simulink subsystem "Kalman_Filter"  (R2019b)
settings: Solver=VariableStepAuto  StartTime=0.0  StopTime=10.0  RelTol=1e-3
undefined symbols (not defined in the file): PF_delay
settings Model: Creator=toons  LastModifiedBy=toons

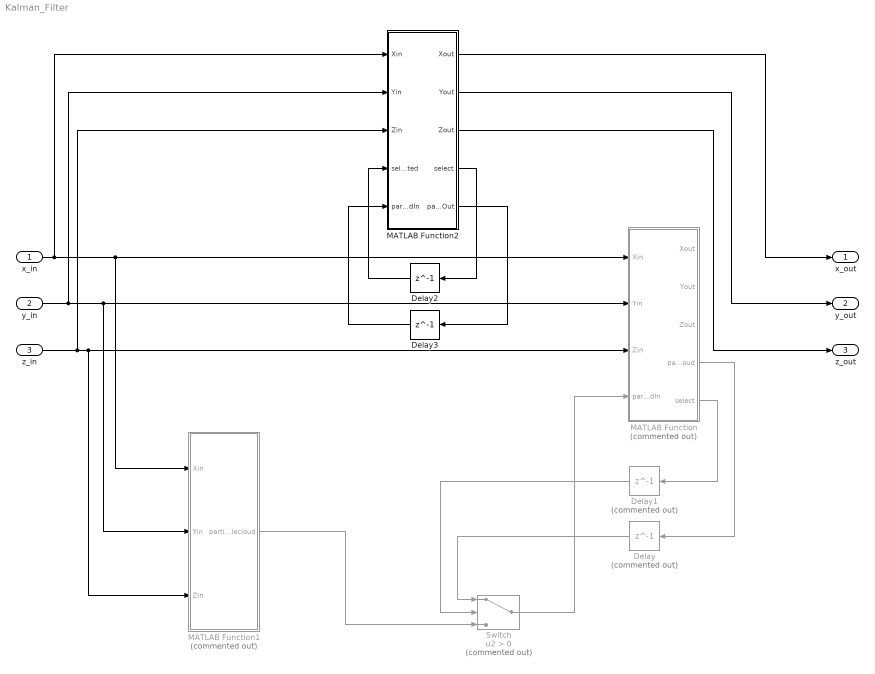
== system Kalman_Filter ==
  x_in : Inport
  y_in : Inport  Port=2
  z_in : Inport  Port=3
  Delay : Delay  Commented=on  DelayLength=1  InitialCondition=0
  Delay1 : Delay  Commented=on  DelayLength=1  InitialCondition=0
  Delay2 : Delay  DelayLength=1  InitialCondition=0  SampleTime=PF_delay
  Delay3 : Delay  DelayLength=1  InitialCondition=0  SampleTime=PF_delay
  MATLAB Function : MATLAB Function  Commented=on  TreatAsAtomicUnit=on
  MATLAB Function1 : MATLAB Function  Commented=on  TreatAsAtomicUnit=on
  MATLAB Function2 : MATLAB Function  TreatAsAtomicUnit=on
  Switch : Switch  Commented=on  Criteria=u2 > Threshold
  x_out : Outport
  y_out : Outport  Port=2
  z_out : Outport  Port=3
  wires:
  y_in/1 -> MATLAB Function1/2(Yin), MATLAB Function/2(Yin), MATLAB Function2/2(Yin)
  x_in/1 -> MATLAB Function1/1(Xin), MATLAB Function/1(Xin), MATLAB Function2/1(Xin)
  z_in/1 -> MATLAB Function1/3(Zin), MATLAB Function/3(Zin), MATLAB Function2/3(Zin)
  MATLAB Function1/1(particlecloud) -> Switch/3
  Switch/1 -> MATLAB Function/4(particlecloudIn)
  MATLAB Function/5(select) -> Delay1/1
  MATLAB Function/4(particlecloud) -> Delay/1
  Delay/1 -> Switch/1
  Delay1/1 -> Switch/2
  MATLAB Function2/1(Xout) -> x_out/1
  MATLAB Function2/2(Yout) -> y_out/1
  MATLAB Function2/3(Zout) -> z_out/1
  MATLAB Function2/4(select) -> Delay2/1
  Delay2/1 -> MATLAB Function2/4(selected)
  MATLAB Function2/5(particlecloudOut) -> Delay3/1
  Delay3/1 -> MATLAB Function2/5(particlecloudIn)

== matlab function Kalman_Filter/MATLAB Function ==
  data: Xin input; Xout output; Yin input; Zin input; Yout output; Zout output; particlecloudIn input; particlecloud output; select output
function [Xout,Yout,Zout, particlecloud, select]= fcn(Xin,Yin,Zin,particlecloudIn)

locationMusquito = [Xin,Yin,Zin];
numberParticles = 500;

xm = locationMusquito(1);
ym = locationMusquito(2);
zm = locationMusquito(3);

measuredPos = locationMusquito;


changeVariationLoc = 0.01;
changeVariationSpeed = 0.01;
changeVariationAngle = 0.4;
changeVariationAcceleration = 0.01;
changeVariationSpeedAngle = 0.1;

particlecloud = particlecloudIn;


    %updateLocation;
    
  particlecloud(:,1) = particlecloud(:,1) + particlecloud(:,4) .* cos(particlecloud(:,5));
  particlecloud(:,2) = particlecloud(:,2) + particlecloud(:,4) .* sin(particlecloud(:,5));
  particlecloud(:,3) = particlecloud(:,3) + particlecloud(:,4) .* sin(particlecloud(:,6));
  particlecloud(:,4) = particlecloud(:,4) + particlecloud(:,7);
  particlecloud(:,5) = particlecloud(:,5) + particlecloud(:,8);
  particlecloud(:,6) = particlecloud(:,6) + particlecloud(:,9);
  particlecloud(:,7) = particlecloud(:,7);
  particlecloud(:,8) = particlecloud(:,8);
  particlecloud(:,9) = particlecloud(:,9);
  
  %L2 difference
  weight = sqrt(measuredPos(1) - particlecloud(:,1)).^2 + (measuredPos(2) - particlecloud(:,2) + (measuredPos(1) - particlecloud(:,1)).^2);
  weight = 1./weight;
  weight = weight ./ sum(weight);
  
  particlecloud(:,24) = particlecloud(:,23);
  particlecloud(:,23) = particlecloud(:,22);
  particlecloud(:,22) = particlecloud(:,21);
  particlecloud(:,21) = particlecloud(:,20);
  particlecloud(:,20) = particlecloud(:,19);
  particlecloud(:,19) = particlecloud(:,18);
  particlecloud(:,18) = particlecloud(:,17);
  particlecloud(:,17) = particlecloud(:,16);
  particlecloud(:,16) = particlecloud(:,15);
  particlecloud(:,15) = particlecloud(:,14);
  particlecloud(:,14) = particlecloud(:,13);
  particlecloud(:,13) = particlecloud(:,12);
  particlecloud(:,12) = particlecloud(:,11);
  particlecloud(:,11) = weight;
  particlecloud(:,10) = (3*particlecloud(:,11)+particlecloud(:,12)+particlecloud(:,13)+particlecloud(:,14)+particlecloud(:,15)+particlecloud(:,16)+particlecloud(:,17)+particlecloud(:,18)+particlecloud(:,19)+particlecloud(:,20)+particlecloud(:,21)+particlecloud(:,22)+particlecloud(:,23)+particlecloud(:,24))./18;
  particlecloud(:,10) = particlecloud(:,10) ./ sum(particlecloud(:,10));
  
  [valueMax indexMax]=max(particlecloud(:,7));
  bestPos = [particlecloud(indexMax,1),particlecloud(indexMax,2), particlecloud(indexMax,3)];
  
  selecting = particlecloud;
  selecting(:,7) = (40*particlecloud(:,8)+particlecloud(:,9)+particlecloud(:,10)+particlecloud(:,11)+particlecloud(:,12)+particlecloud(:,13)+particlecloud(:,14)+particlecloud(:,15)+particlecloud(:,16)+particlecloud(:,17)+particlecloud(:,18)+particlecloud(:,19)+particlecloud(:,20))./14;
  selecting(:,7) = selecting(:,7) ./ sum(selecting(:,7));
  [~,idx] = sort(selecting(:,7)); % sort just the first column
  selecting = selecting(idx,:);   % sort the whole matrix using the sort indices

  for i=1:(numberParticles*0.1)
    particlecloud(i+numberParticles*0.9,:) = selecting(numberParticles-i,:);
  end
  weight = cumsum(weight);
  for i=1:(numberParticles*0.9)
    selecting(i,1) = find(weight >= rand(1),1);
  end
  for i=1:(numberParticles*0.9)
    particlecloud(i,:) = particlecloud(selecting(i,1),:);
        particlecloud(i,1) = particlecloud(i,1) + (rand()*changeVariationLoc - (changeVariationLoc/2));
        particlecloud(i,2) = particlecloud(i,2) + (rand()*changeVariationLoc - (changeVariationLoc/2));
        particlecloud(i,3) = particlecloud(i,3) + (rand()*changeVariationLoc - (changeVariationLoc/2));
        particlecloud(i,4) = particlecloud(i,4) * (rand()*changeVariationSpeed - (changeVariationSpeed/2));
        particlecloud(i,5) = particlecloud(i,5) + (rand()*changeVariationAngle - (changeVariationAngle));
        particlecloud(i,6) = particlecloud(i,6) + (rand()*changeVariationAngle - (changeVariationAngle/2));
        particlecloud(i,7) = particlecloud(i,7) * (rand()*changeVariationAcceleration - (changeVariationAcceleration/2));
        particlecloud(i,8) = particlecloud(i,8) * (rand()*changeVariationSpeedAngle - (changeVariationSpeedAngle/2));
        particlecloud(i,9) = particlecloud(i,9) * (rand()*changeVariationSpeedAngle - (changeVariationSpeedAngle/2));
  end

  select = 1;
Xout = bestPos(1);
Yout = bestPos(2);
Zout = bestPos(3);

== matlab function Kalman_Filter/MATLAB Function1 ==
  data: Xin input; Yin input; Zin input; particlecloud output
function particlecloud = fcn(Xin,Yin,Zin)

locationMusquito = [Xin,Yin,Zin];
numberParticles = 500;

xm = locationMusquito(1);
ym = locationMusquito(2);
zm = locationMusquito(3);

bestPos = locationMusquito;

initialVariationLoc = 0.01;
initialVariationSpeed = 0.01;
initialVariationAngle = 1;
initialVariationAcceleration = 0.01;
initialVariationSpeedAngle = 0.1;

particlecloud = rand(numberParticles,24);

%initial variantion but with avarage zero and then + initial value making
%the initial value the average
particlecloud(:,1) = particlecloud(:,1) * initialVariationLoc - (initialVariationLoc/2) + xm;
particlecloud(:,2) = particlecloud(:,2) * initialVariationLoc - (initialVariationLoc/2) + ym;
particlecloud(:,3) = particlecloud(:,3) * initialVariationLoc - (initialVariationLoc/2) + zm;
% initial variation of speed with zero as the average
particlecloud(:,4) = particlecloud(:,4) * initialVariationSpeed - (initialVariationSpeed/2);
% initial variation of the angle with zero as average
particlecloud(:,5) = particlecloud(:,5) * initialVariationAngle - (initialVariationAngle/2);
particlecloud(:,6) = particlecloud(:,6) * initialVariationAngle - (initialVariationAngle/2);
% initial variation of acceleration with zero as the average
particlecloud(:,7) = particlecloud(:,7) * initialVariationAcceleration - (initialVariationAcceleration/2);
% initial variation of the speed of the angle with zero as average
particlecloud(:,8) = particlecloud(:,8) * initialVariationSpeedAngle - (initialVariationSpeedAngle/2);
particlecloud(:,9) = particlecloud(:,9) * initialVariationSpeedAngle - (initialVariationSpeedAngle/2);
particlecloud(:,10) = 0; % weight
particlecloud(:,11) = 0; % previous weight
particlecloud(:,12) = 0; % the one before and so on
particlecloud(:,13) = 0;
particlecloud(:,14) = 0;
particlecloud(:,15) = 0;
particlecloud(:,16) = 0;
particlecloud(:,17) = 0;
particlecloud(:,18) = 0;
particlecloud(:,19) = 0;
particlecloud(:,20) = 0;
particlecloud(:,21) = 0;
particlecloud(:,22) = 0;
particlecloud(:,23) = 0;
particlecloud(:,24) = 0;

particlecloud = particlecloud;
Xout = bestPos(1);
Yout = bestPos(2);
Zout = bestPos(3);

== matlab function Kalman_Filter/MATLAB Function2 ==
  data: Xin input; Yin input; Zin input; Xout output; selected input; Yout output; Zout output; select output; particlecloudIn input; particlecloudOut output size=[500,24]
function [Xout, Yout, Zout, select, particlecloudOut]= fcn(Xin,Yin,Zin, selected, particlecloudIn)



locationMusquito = [Xin,Yin,Zin];
numberParticles = 500;

particlecloud = rand(numberParticles,24);

particlecloud = particlecloudIn;

xm = locationMusquito(1);
ym = locationMusquito(2);
zm = locationMusquito(3);

bestPos = locationMusquito;

if(selected == 0)

initialVariationLoc = 0.01;
initialVariationSpeed = 0.01;
initialVariationAngle = 1;
initialVariationAcceleration = 0.01;
initialVariationSpeedAngle = 0.1;

particlecloud = rand(numberParticles,24);

%initial variantion but with avarage zero and then + initial value making
%the initial value the average
particlecloud(:,1) = particlecloud(:,1) * initialVariationLoc - (initialVariationLoc/2) + xm;
particlecloud(:,2) = particlecloud(:,2) * initialVariationLoc - (initialVariationLoc/2) + ym;
particlecloud(:,3) = particlecloud(:,3) * initialVariationLoc - (initialVariationLoc/2) + zm;
% initial variation of speed with zero as the average
particlecloud(:,4) = particlecloud(:,4) * initialVariationSpeed - (initialVariationSpeed/2);
% initial variation of the angle with zero as average
particlecloud(:,5) = particlecloud(:,5) * initialVariationAngle - (initialVariationAngle/2);
particlecloud(:,6) = particlecloud(:,6) * initialVariationAngle - (initialVariationAngle/2);
% initial variation of acceleration with zero as the average
particlecloud(:,7) = particlecloud(:,7) * initialVariationAcceleration - (initialVariationAcceleration/2);
% initial variation of the speed of the angle with zero as average
particlecloud(:,8) = particlecloud(:,8) * initialVariationSpeedAngle - (initialVariationSpeedAngle/2);
particlecloud(:,9) = particlecloud(:,9) * initialVariationSpeedAngle - (initialVariationSpeedAngle/2);
particlecloud(:,10) = 0; % weight
particlecloud(:,11) = 0; % previous weight
particlecloud(:,12) = 0; % the one before and so on
particlecloud(:,13) = 0;
particlecloud(:,14) = 0;
particlecloud(:,15) = 0;
particlecloud(:,16) = 0;
particlecloud(:,17) = 0;
particlecloud(:,18) = 0;
particlecloud(:,19) = 0;
particlecloud(:,20) = 0;
particlecloud(:,21) = 0;
particlecloud(:,22) = 0;
particlecloud(:,23) = 0;
particlecloud(:,24) = 0;

particlecloud = particlecloud;


end



measuredPos = locationMusquito;


changeVariationLoc = 0.01;
changeVariationSpeed = 0.01;
changeVariationAngle = 0.4;
changeVariationAcceleration = 0.01;
changeVariationSpeedAngle = 0.1;



    %updateLocation;
    
  particlecloud(:,1) = particlecloud(:,1) + particlecloud(:,4) .* cos(particlecloud(:,5));
  particlecloud(:,2) = particlecloud(:,2) + particlecloud(:,4) .* sin(particlecloud(:,5));
  particlecloud(:,3) = particlecloud(:,3) + particlecloud(:,4) .* sin(particlecloud(:,6));
  particlecloud(:,4) = particlecloud(:,4) + particlecloud(:,7);
  particlecloud(:,5) = particlecloud(:,5) + particlecloud(:,8);
  particlecloud(:,6) = particlecloud(:,6) + particlecloud(:,9);
  particlecloud(:,7) = particlecloud(:,7);
  particlecloud(:,8) = particlecloud(:,8);
  particlecloud(:,9) = particlecloud(:,9);
  
  %L2 difference
  complexweight = sqrt(complex(measuredPos(1) - particlecloud(:,1))).^2 + (measuredPos(2) - particlecloud(:,2) + (measuredPos(1) - particlecloud(:,1)).^2);
  weight = real(complexweight);
  weight = 1./weight;
  weight = weight ./ sum(weight);
  
  particlecloud(:,24) = particlecloud(:,23);
  particlecloud(:,23) = particlecloud(:,22);
  particlecloud(:,22) = particlecloud(:,21);
  particlecloud(:,21) = particlecloud(:,20);
  particlecloud(:,20) = particlecloud(:,19);
  particlecloud(:,19) = particlecloud(:,18);
  particlecloud(:,18) = particlecloud(:,17);
  particlecloud(:,17) = particlecloud(:,16);
  particlecloud(:,16) = particlecloud(:,15);
  particlecloud(:,15) = particlecloud(:,14);
  particlecloud(:,14) = particlecloud(:,13);
  particlecloud(:,13) = particlecloud(:,12);
  particlecloud(:,12) = particlecloud(:,11);
  particlecloud(:,11) = weight;
  particlecloud(:,10) = (3*particlecloud(:,11)+particlecloud(:,12)+particlecloud(:,13)+particlecloud(:,14)+particlecloud(:,15)+particlecloud(:,16)+particlecloud(:,17)+particlecloud(:,18)+particlecloud(:,19)+particlecloud(:,20)+particlecloud(:,21)+particlecloud(:,22)+particlecloud(:,23)+particlecloud(:,24))./18;
  particlecloud(:,10) = particlecloud(:,10) ./ sum(particlecloud(:,10));
  
  [valueMax indexMax]=max(particlecloud(:,7));
  bestPos = [particlecloud(indexMax,1),particlecloud(indexMax,2), particlecloud(indexMax,3)];
  
  selecting = particlecloud;
  selecting(:,7) = (40*particlecloud(:,8)+particlecloud(:,9)+particlecloud(:,10)+particlecloud(:,11)+particlecloud(:,12)+particlecloud(:,13)+particlecloud(:,14)+particlecloud(:,15)+particlecloud(:,16)+particlecloud(:,17)+particlecloud(:,18)+particlecloud(:,19)+particlecloud(:,20))./14;
  selecting(:,7) = selecting(:,7) ./ sum(selecting(:,7));
  [~,idx] = sort(selecting(:,7)); % sort just the first column
  selecting = selecting(idx,:);   % sort the whole matrix using the sort indices

  for i=1:(numberParticles*0.1)
    particlecloud(i+numberParticles*0.9,:) = selecting(numberParticles-i,:);
  end
  weight = cumsum(weight);
  for i=1:(numberParticles*0.9)
      test = find(weight >= rand(1),1);
    selecting(i,1) = test(1,1);
  end
  for i=1:(numberParticles*0.9)
    particlecloud(i,:) = particlecloud(selecting(i,1),:);
        particlecloud(i,1) = particlecloud(i,1) + (rand()*changeVariationLoc - (changeVariationLoc/2));
        particlecloud(i,2) = particlecloud(i,2) + (rand()*changeVariationLoc - (changeVariationLoc/2));
        particlecloud(i,3) = particlecloud(i,3) + (rand()*changeVariationLoc - (changeVariationLoc/2));
        particlecloud(i,4) = particlecloud(i,4) * (rand()*changeVariationSpeed - (changeVariationSpeed/2));
        particlecloud(i,5) = particlecloud(i,5) + (rand()*changeVariationAngle - (changeVariationAngle));
        particlecloud(i,6) = particlecloud(i,6) + (rand()*changeVariationAngle - (changeVariationAngle/2));
        particlecloud(i,7) = particlecloud(i,7) * (rand()*changeVariationAcceleration - (changeVariationAcceleration/2));
        particlecloud(i,8) = particlecloud(i,8) * (rand()*changeVariationSpeedAngle - (changeVariationSpeedAngle/2));
        particlecloud(i,9) = particlecloud(i,9) * (rand()*changeVariationSpeedAngle - (changeVariationSpeedAngle/2));
  end

  select = 1;

Xout = bestPos(1);
Yout = bestPos(2);
Zout = bestPos(3);
particlecloudOut = particlecloud;
